simulink model "aout_eml"  (R2014a)
settings: Solver=FixedStepDiscrete  SolverMode=SingleTasking  StartTime=0.0  StopTime=10.0  RelTol=1e-3
libraries: simulink x1
settings Model: ExtModeTrigDuration=2  Creator=gcampa  LastModifiedBy=gcampa
settings OptimizationCC: OptimizeModelRefInitCode=on  LifeSpan=1
settings DebuggingCC: UnderspecifiedInitializationDetection=Classic  SolverPrmCheckMsg=none  FrameProcessingCompatibilityMsg=error  StateNameClashWarn=warning
settings HardwareCC: ProdBitPerInt=16  ProdBitPerPointer=8  ProdIntDivRoundTo=Zero  ProdEndianess=LittleEndian  ProdWordSize=8  ProdHWDeviceType=Atmel->AVR
settings RTWCC: SystemTargetFile=realtime.tlc  GenerateMakefile=off  TemplateMakefile=realtime.tmf  Description=Run on Target Hardware  RTWVerbose=off  ProcessScript=realtime_make_rtw_hook  CustomSource=..\src\aout_arduino.cpp
settings STFCustomTargetCC: TargetLibSuffix=.a  GenerateSampleERTMain=on  ConcurrentExecutionCompliant=off  GeneratePreprocessorConditionals=Use local settings  ERTCustomFileBanners=on  SupportNonInlinedSFcns=off  SupportVariableSizeSignals=on  MATLABClassNameForMDSCustomization=Simulink.SoftwareTarget.ERTCustomization  GRTInterface=off  SystemTargetFile=realtime.tlc
settings ERTTargetCC: CombineOutputUpdateFcns=off  SupportContinuousTime=on  SupportVariableSizeSignals=on  ExtModeTransport=3  ExtModeMexFile=ext_serial_win32_comm  ExtModeMexArgs=0 1 9600  ERTSrcFileBannerTemplate=realtime_code_template.cgt  ERTHdrFileBannerTemplate=realtime_code_template.cgt  ERTDataSrcFileTemplate=realtime_code_template.cgt  ERTDataHdrFileTemplate=realtime_code_template.cgt  ERTCustomFileTemplate=realtime_file_process.tlc

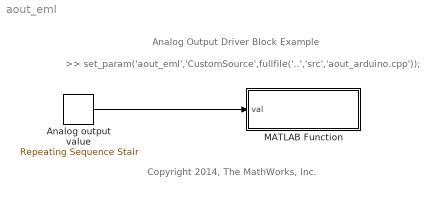
== system aout_eml ==
  note: Analog Output Driver Block Example
  note: Copyright 2014, The MathWorks, Inc.
  note: >> set_param('aout_eml','CustomSource',fullfile('..','src','aout_arduino.cpp'));
  Analog output value : simulink/Sources/Repeating Sequence Stair  OutValues=[20:10:255 255:-10:1]  tsamp=0.01  OutMin=[]  OutMax=[]  OutDataTypeStr=uint8  OutputDataTypeScalingMode=uint8  OutDataType=fixdt(0,8)  ConRadixGroup=Best Precision: Vector-wise  OutScaling=2^-12
  MATLAB Function : MATLAB Function  TreatAsAtomicUnit=on  mask(Analog Write){pin=6, T=0.05}
      mask prompts: T "Sample Time"
      mask help:
      | Every time this block is executed it gets an analog value from 0 or 255 at its input and writes it (via PWM) to a given pin. Basically a square 490Hz waveform is generated with a duty cycle from 0 (corresponding to 0 V) to 255 (corresponding to 5V).
      |
      | The first parameter in the is the number of the pin where the analog output needs to be performed. The second parameter is the sample time.
      |
      | Note that if this block gets copied to a new model, then the file "aout_arduino.cpp" must be added to the CustomSource field of the new model using the "set_param" instruction. See the guide for more info.
  wires:
  Analog output value/1 -> MATLAB Function/1(val)

== matlab function aout_eml/MATLAB Function ==
  settings: updateMethod=DISCRETE  sampleTime=T
  data: pin parameter; val input
function analogWrite(pin,val)
%#codegen

persistent initflag;

if strcmp(coder.target, 'rtw'),
    
    if isempty(initflag),
        % Initialize step
        coder.ceval('aout_init',uint8(pin));
        initflag = 1;
    else
        % output Step
        coder.ceval('aout_output', uint8(pin), uint8(val));
    end
    
end
